simulink model "full_3omni_ctrl_sim_and_exp_with_xpctarget"  (R2014b)
settings: Solver=ode3  SolverMode=SingleTasking  StartTime=0.0  StopTime=40  FixedStep=0.01  RelTol=1e-3
libraries: xpcobsoletelib x13, simulink x10, xpcutilitieslib x3, slrtlib x3
(part 2 of 2)

== stateflow chart full_3omni_ctrl_sim_and_exp_with_xpctarget/Manual and auto designer ==
  state Initialization
    entry:
    totalPpr = 60*ones(6,1);
    gearRatio = 19.2*ones(6,1);
    drivPwmFreq = 400; % Hz
    genPwmFreq = 80e6; % Hz
    battVol = 18.4;
    vMax = 2;
    accel = 0.5;
    omegaMax = 1;
    angAccel = 0.3;
    opMode = manual;
    t_dep = [0;0];
    departPose = Xd;
    terminalPose = Xd;
    [isUpdate,Xr] = wayPoints(...
    manual,xytheta,Xd);
    i_max = length(Xr(1,:));
    j_max = i_max;
  state Manual
    entry:
    t_dep = [t;t]; i1 = 1;
    departPose = Xd;
    during:
    [isUpdate,Xr] = wayPoints(manual,xytheta,Xd);
    terminalPose = Xr(:,1);
    if detectChange
    departPose = Xd;
    terminalPose = Xd
    end
  state Semi_autonomous
    entry: [isUpdate,Xr] = wayPoints(manual,xytheta,Xd);
    state Autonomous1
      during:
      if norm(Xr(1:2,i)-Xd(1:2)) < 0.15 && i < i_max
      departPose(1:2) = Xd(1:2);
      terminalPose(1:2) = Xr(1:2,i+1);
      i = i+1;
      t_dep(1) = t;
      end
      if abs(Xr(3,j)-Xd(3)) <  0.05 && j < j_max
      departPose(3) = Xd(3);
      terminalPose(3) = Xr(3,j+1);
      j = j+1;
      t_dep(2) = t;
      end
    state Autonomous
      entry:
      t_dep = [t;t];
      departPose = Xd;
      terminalPose = Xr(:,1);
      i = 1; j = 1;
    (default) -> Autonomous
    Autonomous1 -> Autonomous : [isUpdate]
    Autonomous -> Autonomous1 : [~isUpdate]
  (junction 18) -> (junction 14) : [start && ~manual]
  (default) -> Initialization
  Initialization -> (junction 18) [order 2]
  (junction 14) -> Semi_autonomous
  Initialization -> Manual [order 1] : [manual]
  Manual -> Semi_autonomous : [start && ~manual]
  Semi_autonomous -> Manual : [detectChange]
  data: update function_output; Xp function_output; op function_input; xyo function_input; Xdes function_input; opMode output; totalPpr output; gearRatio output; drivPwmFreq output; genPwmFreq output; battVol output; manual input; xytheta input size=2; detectChange input; t input; start input; Xd_dot input; Xd input; t_dep output; vMax output; accel output; omegaMax output; angAccel output; terminalPose output; departPose output; j_max local; j local; i local; i_max local; i1 local; Xr local size=[3,20]; isUpdate local
  function [update,Xp] = wayPoints(op,xyo,Xdes):
    | function [update,Xp] = wayPoints(op,xyo,Xdes)
    | 
    | persistent X
    | if isempty(X), X = zeros(3,1);end
    | Xp = zeros(3,20);
    |  update = 0;
    | % %Maximum number of column of X is 20
    | 
    | if op
    |     update = 1;
    |     if xyo(1)==2
    |         X(1,1) = 100;
    |     elseif xyo(1)==4
    |         X(1,1) = -100;
    |     elseif xyo(1)==1
    |         X(2,1) = 100;
    |     elseif xyo(1)==3
    |         X(2,1) = -100;
    |     elseif xyo(2)==5
    |         X(3,1) = 100;
    |     elseif xyo(2)==6
    |         X(3,1) = -100;
    |     else
    |         X = Xdes;
    |     end
    | else
    |     X = [
    |     1   4   2.5 6
    |     2   2.5 3   4
    |     1   3   2   3.5
    |     ];
    | end
    | nPoints = length(X(1,:));
    | Xp(:,1:nPoints) = X;
    | Xp(:,nPoints+1:20) = repmat(X(:,nPoints),1,20-nPoints);

== matlab function full_3omni_ctrl_sim_and_exp_with_xpctarget/Identification/MATLAB Function1 ==
  data: x_hat input; KnTau output
function KnTau = fcn(x_hat)

KnTau = [x_hat(3)/x_hat(2); 1/x_hat(2)];

== matlab function full_3omni_ctrl_sim_and_exp_with_xpctarget/Simulation/Friction ==
  data: w input; vf output
function vf = fcn(w)

vf = 0.13*sigmoidFcn(w);
end

function y = sigmoidFcn(x)
y = 2./(1+exp(-15*x))-1; % element wise computing
end

== matlab function full_3omni_ctrl_sim_and_exp_with_xpctarget/Kinematics for 3 omni wheels/Forward Kinematics ==
  data: fi_dot input; x_dot output
function x_dot = fcn(fi_dot)

R = 0.064044; % Radius of omni directional wheel
L = 0.3113;  % Radius of MR1


% x_dot = R*[(cos(theta - pi/3) - cos(pi/3 + theta))/(cos(theta)*sin(theta - pi/3) - cos(theta)*sin(pi/3 + theta) - cos(theta - pi/3)*sin(theta) + cos(pi/3 + theta)*sin(theta) - cos(theta - pi/3)*sin(pi/3 + theta) + cos(pi/3 + theta)*sin(theta - pi/3)),(cos(theta) + cos(pi/3 + theta))/(cos(theta)*sin(theta - pi/3) - cos(theta)*sin(pi/3 + theta) - cos(theta - pi/3)*sin(theta) + cos(pi/3 + theta)*sin(theta) - cos(theta - pi/3)*sin(pi/3 + theta) + cos(pi/3 + theta)*sin(theta - pi/3)),-(cos(theta) + cos(theta - pi/3))/(cos(theta)*sin(theta - pi/3) - cos(theta)*sin(pi/3 + theta) - cos(theta - pi/3)*sin(theta) + cos(pi/3 + theta)*sin(theta) - cos(theta - pi/3)*sin(pi/3 + theta) + cos(pi/3 + theta)*sin(theta - pi/3))
%   (sin(theta - pi/3) - sin(pi/3 + theta))/(cos(theta)*sin(theta - pi/3) - cos(theta)*sin(pi/3 + theta) - cos(theta - pi/3)*sin(theta) + cos(pi/3 + theta)*sin(theta) - cos(theta - pi/3)*sin(pi/3 + theta) + cos(pi/3 + theta)*sin(theta - pi/3)),(sin(theta) + sin(pi/3 + theta))/(cos(theta)*sin(theta - pi/3) - cos(theta)*sin(pi/3 + theta) - cos(theta - pi/3)*sin(theta) + cos(pi/3 + theta)*sin(theta) - cos(theta - pi/3)*sin(pi/3 + theta) + cos(pi/3 + theta)*sin(theta - pi/3)),-(sin(theta) + sin(theta - pi/3))/(cos(theta)*sin(theta - pi/3) - cos(theta)*sin(pi/3 + theta) - cos(theta - pi/3)*sin(theta) + cos(pi/3 + theta)*sin(theta) - cos(theta - pi/3)*sin(pi/3 + theta) + cos(pi/3 + theta)*sin(theta - pi/3))
%  -(cos(theta - pi/3)*sin(pi/3 + theta) - cos(pi/3 + theta)*sin(theta - pi/3))/(L*cos(theta)*sin(theta - pi/3) - L*cos(theta)*sin(pi/3 + theta) - L*cos(theta - pi/3)*sin(theta) + L*cos(pi/3 + theta)*sin(theta) - L*cos(theta - pi/3)*sin(pi/3 + theta) + L*cos(pi/3 + theta)*sin(theta - pi/3)),-(cos(theta)*sin(pi/3 + theta) - cos(pi/3 + theta)*sin(theta))/(L*cos(theta)*sin(theta - pi/3) - L*cos(theta)*sin(pi/3 + theta) - L*cos(theta - pi/3)*sin(theta) + L*cos(pi/3 + theta)*sin(theta) - L*cos(theta - pi/3)*sin(pi/3 + theta) + L*cos(pi/3 + theta)*sin(theta - pi/3)),(cos(theta)*sin(theta - pi/3) - cos(theta - pi/3)*sin(theta))/(L*cos(theta)*sin(theta - pi/3) - L*cos(theta)*sin(pi/3 + theta) - L*cos(theta - pi/3)*sin(theta) + L*cos(pi/3 + theta)*sin(theta) - L*cos(theta - pi/3)*sin(pi/3 + theta) + L*cos(pi/3 + theta)*sin(theta - pi/3))]*fi_dot;

x_dot = R*[0, -sqrt(3)/3, sqrt(3)/3
          2/3,   -1/3,     -1/3
         1/(3*L) 1/(3*L)  1/(3*L)]*fi_dot;
    
% x_dot=R*(-2/3*sin(theta)*w1-2/3*sin(pi/3-theta)*w2+2/3*sin(pi/3+theta)*w3);
% y_dot=R*(2/3*cos(theta)*w12-2/3*cos(pi/3-theta)*w2-2/3*cos(pi/3+theta)*w3);
% theta_dot=R*(1/3*L)*w1+(1/3*L)*w2+(1/3*L)*w3;

% x_dot=[x_dot;y_dot;theta_dot];
% x_dot(1)=x_dot;
% x_dot(2)=y_dot;
% x_dot(3) = theta_dot;

== matlab function full_3omni_ctrl_sim_and_exp_with_xpctarget/Kinematics for 3 omni wheels/Inverse Kinematics1 ==
  data: thetad input; u input; fi_dot output
function fi_dot  = fcn(thetad,u)

%R = 0.064044; % Radius of omni directional wheel
%L = 0.3113;  % Radius of MR1
L_R = 4.8607;
R = 0.061;
L = L_R*R;

fi_dot = (1/R)*[-sin(thetad) cos(thetad) L
    -sin(pi/3-thetad) -cos(pi/3-thetad) L
    sin(pi/3+thetad) -cos(pi/3+thetad) L]*u;

% w2=(1/R)*(-x_dot*sin(pi/3-theta)+y_dot*cos(pi/3-theta)+L*theta_dot);
% w3=(1/R)*(-x_dot*sin(theta+pi/3)+y_dot*cos(theta+pi/3)+L*theta_dot);
% 
% fi_dot=[w1;w2;w3];
% fi_dot(1)=w1;
% fi_dot(2)=w2;
% fi_dot(3)=w3;

== matlab function full_3omni_ctrl_sim_and_exp_with_xpctarget/Kinematics for 3 omni wheels/Trajectory velocity generation ==
  data: t input; X_r_dot output; t_dep input; Vmax input; accel input; omegaMax input; angAccel input; terminalPose input; departPose input
function X_r_dot = fcn(t,t_dep,Vmax,accel,omegaMax,angAccel,terminalPose,departPose)
%#codegen

Vmax = abs(Vmax); omegaMax = abs(omegaMax);
if Vmax == 0
    Vmax = 1e-5;
end
if omegaMax ==0
    omegaMax = 1e-5;
end
% Vmax = 4; % maximum velocity
%accel = 0.5;      % acceleration
% omegaMax = 3;
%angAccel = 0.7;

X_r_dot = zeros(3,1);


dX = terminalPose(1:2)-departPose(1:2);
norm_dX = norm(dX);
two_rmin = Vmax^2/accel;
dtheta = terminalPose(3)-departPose(3);
norm_dtheta = abs(dtheta);
two_thetamin = omegaMax^2/angAccel;

if norm_dX > two_rmin
    ta = Vmax/accel;                   % acceleration period
    tad = (norm_dX-two_rmin)/Vmax; % acc to deceleration period
    td = ta + tad;                  % start deceleration
    te = ta + td;                   % end deceleration
    if (t-t_dep(1)) < ta
        speed = accel*(t-t_dep(1));
    elseif ta <= (t-t_dep(1)) && (t-t_dep(1)) < td
        speed = Vmax;
    elseif td <= (t-t_dep(1)) && (t-t_dep(1)) < te
        speed = -accel*(t-t_dep(1)-td) + Vmax;
    else
        speed = 0;
    end
else
    tp = sqrt(norm_dX/accel);
    te = 2*tp;
    Vp = accel*tp;
    if (t-t_dep(1)) < tp
        speed = accel*(t-t_dep(1));
    elseif tp <= (t-t_dep(1)) && (t-t_dep(1)) < te
        speed = -accel*(t-t_dep(1)-tp)+Vp;
    else
        speed = 0;
    end
end
if norm_dX~=0
    X_r_dot(1:2) = speed*dX/norm_dX;
end

if norm_dtheta > two_thetamin
    ta = omegaMax/angAccel;                   % acceleration period
    tad = (norm_dtheta-two_thetamin)/omegaMax; % acc to deceleration period
    td = ta + tad;                  % start deceleration
    te = ta + td;                   % end deceleration
    if (t-t_dep(2)) < ta
        omegaSpeed = angAccel*(t-t_dep(2));
    elseif ta <= (t-t_dep(2)) && (t-t_dep(2)) < td
        omegaSpeed = omegaMax;
    elseif td <= (t-t_dep(2)) && (t-t_dep(2)) < te
        omegaSpeed = -angAccel*(t-t_dep(2)-td) + omegaMax;
    else
        omegaSpeed = 0;
    end
else
    tp = sqrt(norm_dtheta/angAccel);
    te = 2*tp;
    omegap = angAccel*tp;
    if (t-t_dep(2)) < tp
        omegaSpeed = angAccel*(t-t_dep(2));
    elseif tp <= (t-t_dep(2)) && (t-t_dep(2)) < te
        omegaSpeed = -angAccel*(t-t_dep(2)-tp)+omegap;
    else
        omegaSpeed = 0;
    end
end
X_r_dot(3) = omegaSpeed*sign(dtheta);

== matlab function full_3omni_ctrl_sim_and_exp_with_xpctarget/Kinematics for 3 omni wheels/Rotation Matrix (R(theta)) ==
  data: theta input; X_w_dot output; X_R_dot input
function X_w_dot = fcn(theta,X_R_dot)
%#codegen

R = [cos(theta) -sin(theta) 0; sin(theta) cos(theta) 0; 0 0 1];
X_w_dot = R*X_R_dot;

== stateflow chart full_3omni_ctrl_sim_and_exp_with_xpctarget/Identification/Chart2 ==
  state IdentifyKTauFr
    entry:
    %A = [W_ave ones(16,1)];
    %KbRiKtauFr(1:2) = (A'*A)\A'*V;
    %KbRiKtauFr(3) = 1/KbRiKtauFr(1);
    T = 0; t_ref = t; i = 1;
    a_ave = x_hat(2); b_ave = x_hat(3);
    c_ave = x_hat(4);
    during:
    T = t - t_ref; offset = 0;
    Va = (battVol-3 - offset)*sin(2*T)+offset;
    x_hat = UKF(Va,w_measure,dt);
    if T<10*Th
    a_ave = x_hat(2); b_ave = x_hat(3);
    c_ave = x_hat(4);
    else
    a_ave = (a_ave*i + x_hat(2))/(i+1);
    b_ave = (b_ave*i + x_hat(3))/(i+1);
    c_ave = (c_ave*i + x_hat(4))/(i+1);
    i = i+1;
    end
    exit:
    KbRiKtauFr(3) = b_ave/a_ave;
    KbRiKtauFr(4) = 1/a_ave;
    KbRiKtauFr(5) = c_ave/b_ave;
  state Resting
    entry: T = 0; t_ref = t; Va = 0;
    during: T = t - t_ref;
  state Initialization
    entry:
    Va = 2;
    Vinc = 1;
    Th = 1;
    n = 0;
    n_max = 16;
    dt = 0.01;
    w_ave = 0;
    W_ave = zeros(16,1);
    V = W_ave;
    KbRiKtauFr = 0.1*ones(5,1);
    controller = [0;0;0];
    t_contr = 0;
    posError = 0;
    x_hat = 0.1*ones(4,1);
  state VoltageIncrement [commented out]
    entry:
    t_ref = t;
    n = n+1; T = 0;
    if n<n_max/2 + 2
    Va = Va+Vinc;
    else
    Va = Va-Vinc;
    end
    during:
    T = t - t_ref;
  state FeedbackControl
    entry:
    t_ref = t; pos_ref = measuredPos;
    K = KbRiKtauFr(3); tau = KbRiKtauFr(4);
    z = 1.45*a_ave;
    Kd = 1*(2*(tau*z+sqrt(tau*z*(tau*z-1)))-1)/K;
    controller(1) = Kd*z; controller(2) = 0;
    controller(3) = Kd;
    during:
    t_contr = t - t_ref;
    posError = desiredPos - ...
    measuredPos + pos_ref;
    Va = PID(posError,controller,K,battVol,dt) ...
    + desiredVel;
    Va = Va/K+ c_ave/b_ave*sign(desiredVel);
  state AveragingInputOutput [commented out]
    entry:
    i = 1;
    w_ave = w_measure;
    during:
    w_ave = (w_ave*i + w_measure)/(i+1);
    i = i+1; T = t - t_ref;
    exit:
    W_ave(n) = w_ave; V(n) = Va;
  IdentifyKTauFr -> Resting : [T>20*Th]
  Initialization -> IdentifyKTauFr : [1]
  (default) -> Initialization
  Resting -> FeedbackControl : [T>2*Th]
  Initialization -> VoltageIncrement [commented out] : [1]
  VoltageIncrement -> IdentifyKTauFr [commented out] : [n>n_max]
  VoltageIncrement -> AveragingInputOutput [commented out] : [T>Th]
  AveragingInputOutput -> VoltageIncrement [commented out] : [T>2*Th]
  data: err function_input; u function_output; contr function_input; gain function_input; limit function_input; Ts function_input; u_ function_input; y_meas function_input; x function_output; Ts function_input; t_contr output; KbRiKtauFr output size=5; controller output size=3; t input; w_measure input; desiredVel input; desiredPos input; n local; n_max local; Vinc local; Th local; A local size=[16,2]; i local; t_ref local; offset local; a_ave local; b_ave local; measuredPos input; tau local; z local; Kd local; K local; pos_ref local; posError output; x_hat output size=4; T local; dt local; c_ave local; W_ave local size=16; V local size=16; w_ave output; Va output; battVol input
  function u = PID(err,contr,gain,limit,Ts):
    | function u = PID(err,contr,gain,limit,Ts)
    | 
    | persistent integrator;
    | persistent differentiator;
    | persistent err_d1;
    | if isempty(integrator)
    |     integrator = 0;
    |     differentiator = 0;
    |     err_d1 = 0;
    | end
    | tau = 0.04;
    | contr = contr*gain;
    | kp = contr(1); ki = contr(2); kd = contr(3);
    | integrator = integrator + (Ts/2)*(err + err_d1);
    |  % update integrator
    |  differentiator = (2*tau-Ts)/(2*tau+Ts)*differentiator...
    |  + 2/(2*tau+Ts)*(err - err_d1);
    |  % update differentiator
    |  err_d1 = err; % update the err for next time through
    |  % the loop
    |  u = sat(... % implement PID control
    |  kp * err +... % proportional term
    |  ki * integrator +... % integral term
    |  kd * differentiator,... % derivative term
    |  limit... % ensure abs(u)<=limit
    |  );
    |  % implement integrator antiwindup
    |  if ki~=0
    |  u_unsat = kp*err + ki*integrator + kd*differentiator;
    |  integrator = integrator + Ts/ki * (u - u_unsat);
    |  end
    | end
    | function u_sat = sat(value,limit)
    | if value < -limit
    |     u_sat = -limit;
    | elseif value > limit
    |     u_sat = limit;
    | else
    |     u_sat = value;
    | end
    | end
  function x = UKF(u_,y_meas,Ts):
    | function x = UKF(u_,y_meas,Ts)
    | 
    | n = 4;
    | m = 1;
    | Q = 1e-5*diag([1 1000 10000 1000]);
    | R = 1e-2;
    | 
    | nSigma = 2*4+1;
    | 
    | persistent x_ P_ wm W lambda
    | if isempty(x_)
    |     x_= 0.1*ones(4,1); P_ = 1e-1*eye(4);
    |     k=2;
    |     alpha=0.5; beta=1;
    |     lambda=alpha^2*(n+k)-n;
    |     Wm0=lambda/(n+lambda);
    |     Wc0=lambda/((n+lambda)+(1-alpha^2+beta));
    |     Wmi=1/2/(n+lambda);
    |     Wci=Wmi;
    |     wm=Wmi*ones(nSigma,1); wm(1)=Wm0;
    |     W=(eye(nSigma)-wm*ones(1,nSigma))...
    |      *diag([Wc0 Wci*ones(1,2*4)])...
    |      *(eye(nSigma)-wm*ones(1,nSigma))';
    | end
    | 
    | sqrtP = chol(P_,'lower');
    | X_= x_*ones(1,nSigma) + ...
    |         sqrt(n+lambda)*[zeros(4,1) sqrtP -sqrtP];
    | X = X_;
    | for i=1:nSigma
    |     X(:,i)= fd(X_(:,i),u_,Ts);
    | end
    | x1     = X*wm;
    | x = x1(1:4,1);
    | P     = X*W*X'+Q;
    | 
    | %Measurement Update
    | %Re-Generate Sigma Points
    | sqrtP   = chol(P,'lower');
    | X   = x*ones(1,nSigma) + ...
    |         sqrt(n+lambda)*[zeros(4,1) sqrtP -sqrtP];
    | Y   = zeros(m,nSigma);
    | for i=1:nSigma
    |     Y(:,i)= hd(X(:,i));
    | end
    | y   = Y*wm;
    | Pxy = X*W*Y';
    | Pyy = Y*W*Y'+R;
    | KK   = Pxy/Pyy;
    | x_  = x + KK*(y_meas-y);
    | P_  = P - KK*Pyy*KK';
    | 
    | end
    | 
    | function x = fd(x_,u_,Ts)
    | % w_dot = -a*w + b*u - c*sign(w)
    | 
    | % Let x(1)=w, x(2)=a, x(3)=b, x(4)=c, then
    | % x_dot(1) = -x(1)*x(2) + x(3)*u - x(4)*sign(x(1))
    | % x_dot(2) = 0    (since a is constant)
    | % x_dot(3) = 0    (since b is constant)
    | % x_dot(4) = 0    (since c is constant)
    | % In compact form
    | % x_dot = f(x,u)
    | 
    | % Rewritten in discrete form as
    | % x(k) = x(k-1) + f(x(k-1),u(k-1))*Ts
    | 
    | x = x_ + [-x_(1)*x_(2)+x_(3)*u_-x_(4)*sigmoidFcn(x_(1));0;0;0]*Ts;
    | end
    | 
    | function y = hd(x)
    | C = [1 0 0 0];
    | y = C*x;
    | end
    | 
    | function y = sigmoidFcn(x)
    | y = 2/(1+exp(-20*x))-1;
    | end

== matlab function full_3omni_ctrl_sim_and_exp_with_xpctarget/Kinematics for 3 omni wheels/MATLAB Function1 ==
  settings: updateMethod=DISCRETE
  data: Ts output; t input; t_dep input; omegaMax input; omega output; terminalPose input; departPose input
function [Ts,omega] = fcn(t,t_dep,omegaMax,terminalPose,departPose)
%#codegen

persistent  t1
if isempty(t1)
    t1 = 0;
end

Ts = t-t1;
t1 = t;
omegaMax = abs(omegaMax);
if omegaMax == 0
    omegaMax = 1e-5;
end
angAccel = 0.5;

dtheta = terminalPose-departPose;
norm_dtheta = abs(dtheta);
two_thetamin = omegaMax^2/angAccel;

if norm_dtheta > two_thetamin
    ta = omegaMax/angAccel;                   % acceleration period
    tad = (norm_dtheta-two_thetamin)/omegaMax; % acc to deceleration period
    td = ta + tad;                  % start deceleration
    te = ta + td;                   % end deceleration
    if (t-t_dep) < ta
        omega = angAccel*(t-t_dep);
    elseif ta <= (t-t_dep) && (t-t_dep) < td
        omega = omegaMax;
    elseif td <= (t-t_dep) && (t-t_dep) < te
        omega = -angAccel*(t-t_dep-td) + omegaMax;
    else
        omega = 0;
    end
else
    tp = sqrt(norm_dtheta/angAccel);
    te = 2*tp;
    omegap = angAccel*tp;
    if (t-t_dep) < tp
        omega = angAccel*(t-t_dep);
    elseif tp <= (t-t_dep) && (t-t_dep) <= te
        omega = -angAccel*(t-t_dep-tp)+omegap;
    else
        omega = 0;
    end
end
omega = omega*sign(dtheta);

== stateflow chart full_3omni_ctrl_sim_and_exp_with_xpctarget/Kinematics for 3 omni wheels/Chart ==
  state Initialization
    entry:
    t_dep = t;
    omegaMax = 0.5;
    terminalPose = theta_d;
    departPose = theta_d;
  state Kick
    entry:
    t_dep = t;
    departPose = theta_d;
    terminalPose = terminalPose + 2*pi;
  (default) -> Initialization
  Initialization -> Kick : [kick]
  Kick -> Initialization : [abs(terminalPose - theta_d) < pi/360]
  data: t input; t_dep output; omegaMax output; terminalPose output; kick input; theta_d input; departPose output
